simulink model "ECM"  (R2021b)
settings: Solver=VariableStepAuto  StartTime=0.0  StopTime=time(end)  RelTol=1e-3
values from neighbouring files (symbols this model uses):
  LookUpTables = struct    [LUT.m]    (also in Run_parameterestimation.m = load([Rep_Meatech, filesep,'LookUpTables_HPPC.mat']); Script_SOC_EKF.m = load('LookUpTables.mat'))
  Qnom = 2.455    [Pulse_extraction.m]    (also in Script_validation.m = 2.4162)
  SOC_init = 100    [Pulse_extraction.m]    (also in Script_SOC_EKF.m; Script_validation.m = 50)
  T_init = meas.Battery_Temp_degC(1)    [Script_validation.m]
libraries: simulink x4
settings Model: Creator=joel-louis.kone  LastModifiedBy=joel-louiskone
settings SolverCC: AlgebraicLoopSolver=TrustRegion
settings DebuggingCC: UnconnectedInputMsg=none  UnconnectedOutputMsg=none  UnconnectedLineMsg=none  SFMachineParentedDataDiag=warning
settings ModelReferenceCC: EnableRefExpFcnMdlSchedulingChecks=off

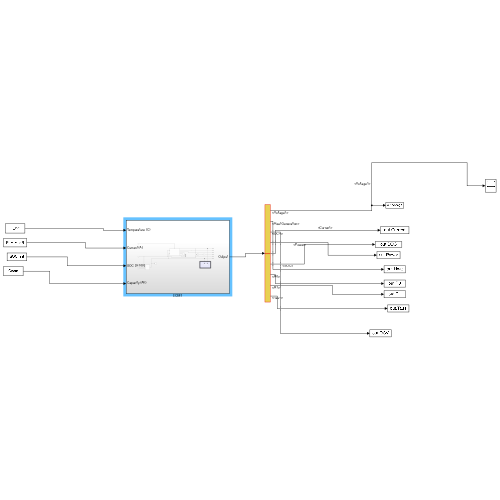
[thumbnail: Simulink's stored preview of the top-level diagram]
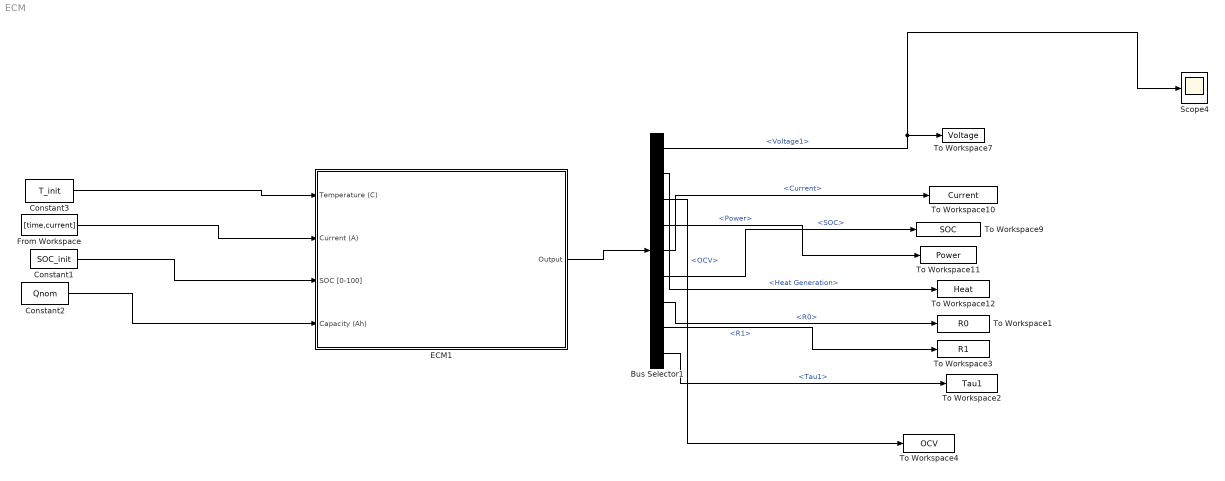
== system ECM ==
  Bus Selector1 : BusSelector  OutputSignals=Voltage1,Heat Generation,OCV,Power,Current,SOC,R0,R1,Tau1
  Constant1 : Constant  Value=SOC_init
  Constant2 : Constant  Value=Qnom
  Constant3 : Constant  Value=T_init
  ECM1 : Subsystem
  From Workspace : FromWorkspace  VariableName=[time,current]  SampleTime=0.1
  Scope4 : Scope
  To Workspace1 : ToWorkspace  VariableName=R0  SaveFormat=Structure With Time  SampleTime=-1
  To Workspace10 : ToWorkspace  VariableName=Current  SaveFormat=Structure With Time  SampleTime=-1
  To Workspace11 : ToWorkspace  VariableName=Power  SaveFormat=Structure With Time  SampleTime=-1
  To Workspace12 : ToWorkspace  VariableName=Heat  SaveFormat=Structure With Time  SampleTime=-1
  To Workspace2 : ToWorkspace  VariableName=Tau1  SaveFormat=Structure With Time  SampleTime=-1
  To Workspace3 : ToWorkspace  VariableName=R1  SaveFormat=Structure With Time  SampleTime=-1
  To Workspace4 : ToWorkspace  VariableName=OCV  SaveFormat=Structure With Time  SampleTime=-1
  To Workspace7 : ToWorkspace  VariableName=Voltage  SaveFormat=Structure With Time  SampleTime=-1
  To Workspace9 : ToWorkspace  VariableName=SOC  SaveFormat=Structure With Time  SampleTime=-1
  wires:
  Bus Selector1/5 -> To Workspace10/1  "<Current>"
  From Workspace/1 -> ECM1/2(Current (A))
  Bus Selector1/2 -> To Workspace12/1  "<Heat Generation>"
  Constant3/1 -> ECM1/1(Temperature (C))
  ECM1/1(Output) -> Bus Selector1/1
  Bus Selector1/1 -> Scope4/1, To Workspace7/1  "<Voltage1>"
  Bus Selector1/6 -> To Workspace9/1  "<SOC>"
  Bus Selector1/4 -> To Workspace11/1  "<Power>"
  Constant2/1 -> ECM1/4(Capacity (Ah))
  Constant1/1 -> ECM1/3(SOC [0-100])
  Bus Selector1/7 -> To Workspace1/1  "<R0>"
  Bus Selector1/8 -> To Workspace3/1  "<R1>"
  Bus Selector1/9 -> To Workspace2/1  "<Tau1>"
  Bus Selector1/3 -> To Workspace4/1  "<OCV>"

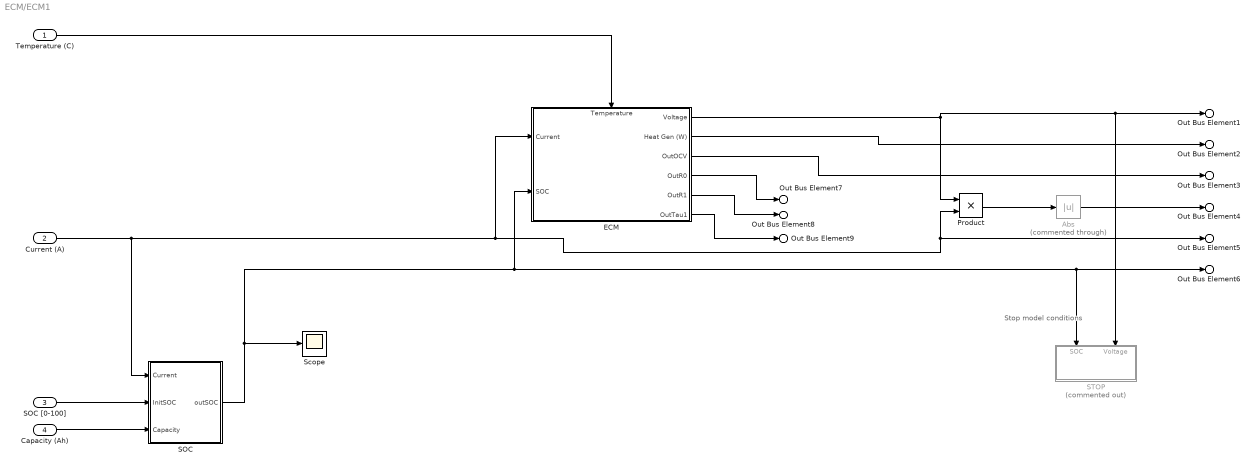
== system ECM/ECM1 ==
  note: Stop model conditions
  Temperature (C) : Inport
  Current (A) : Inport  Port=2
  SOC [0-100] : Inport  Port=3
  Capacity (Ah) : Inport  Port=4
  Abs : Abs  Commented=through
  ECM : Subsystem
      settings: PortSchema="{\"entries\":[{\"content\":{\"sides\":[{\"content\":{\"connectorIds\":[\"In1\",\"In2\"]},\"type\":\"ConnectorPlacement.EquallySpacedRectSide\",\"uuid\":\"edc5e7ae-745c-47cf-82e1-2a35e82af4f8\"},{\"content\":{\"connectorIds\":[\"Out1\",\"Out2\",\"Out3\",\"Out4\",\"Out5\",\"Out6\"],\"side\":\"RIGHT\"},\"type\":\"ConnectorPlacement.EquallySpacedRectSide\",\"uuid\":\"23604a62-cf3d-4676-b110-c126866d2dc0\"},{\"content\":{\"connectorIds\":[\"In3\"],\"side\":\"TOP\"},\"type\":\"ConnectorPlacement.EquallySpacedRectSide\",\"uuid\":\"e8176ec1-85b7-4cdd-8c72-13c05cb96821\"}]},\"type\":\"ConnectorPlacement.EquallySpacedConnector\",\"uuid\":\"8076f895-f62a-482c-9288-582d3af41eba\"}],\"packageUris\":[\"http://schema.mathworks.com/mf0/Connector/R2020b\"],\"version\":\"1.0\"}"
  Product : Product
  SOC : Subsystem
  STOP : Subsystem  Commented=on
      settings: PortSchema="{\"entries\":[{\"content\":{\"sides\":[{\"content\":{},\"type\":\"ConnectorPlacement.EquallySpacedRectSide\",\"uuid\":\"ad4b06f7-1952-4c9b-98d0-1c5b14fc528a\"},{\"content\":{\"side\":\"RIGHT\"},\"type\":\"ConnectorPlacement.EquallySpacedRectSide\",\"uuid\":\"0e87e05f-c38b-4899-9ed0-4e84cd23c8de\"},{\"content\":{\"side\":\"TOP\"},\"type\":\"ConnectorPlacement.EquallySpacedRectSide\",\"uuid\":\"e38574cc-e4d8-43c2-a247-2bbd6f40e998\"},{\"content\":{\"connectorIds\":[\"In1\",\"In2\"],\"side\":\"BOTTOM\"},\"type\":\"ConnectorPlacement.EquallySpacedRectSide\",\"uuid\":\"fa834913-df18-4dba-ad85-ee110dbadbfc\"}]},\"type\":\"ConnectorPlacement.EquallySpacedConnector\",\"uuid\":\"cbbb9c3f-18ca-424a-bd7b-42dc7388afb6\"}],\"packageUris\":[\"http://schema.mathworks.com/mf0/Connector/R2020b\"],\"version\":\"1.0\"}"
  Scope : Scope
  Out Bus Element1 : Outport  PortName=Output  Element=Voltage1
  Out Bus Element2 : Outport  PortName=Output  Element=Heat Generation
  Out Bus Element3 : Outport  PortName=Output  Element=OCV
  Out Bus Element4 : Outport  PortName=Output  Element=Power
  Out Bus Element5 : Outport  PortName=Output  Element=Current
  Out Bus Element6 : Outport  PortName=Output  Element=SOC
  Out Bus Element7 : Outport  PortName=Output  Element=R0
  Out Bus Element8 : Outport  PortName=Output  Element=R1
  Out Bus Element9 : Outport  PortName=Output  Element=Tau1
  wires:
  SOC [0-100]/1 -> SOC/2(InitSOC)
  Current (A)/1 -> Product/2, Out Bus Element5/1, ECM/1(Current), SOC/1(Current)
  ECM/2(Heat Gen (W)) -> Out Bus Element2/1
  ECM/1(Voltage) -> Product/1, Out Bus Element1/1, STOP/1(Voltage)
  Capacity (Ah)/1 -> SOC/3(Capacity)
  ECM/3(OutOCV) -> Out Bus Element3/1
  Product/1 -> Abs/1
  Abs/1 -> Out Bus Element4/1
  Temperature (C)/1 -> ECM/3(Temperature)
  SOC/1(outSOC) -> Out Bus Element6/1, STOP/2(SOC), ECM/2(SOC), Scope/1
  ECM/4(OutR0) -> Out Bus Element7/1
  ECM/5(OutR1) -> Out Bus Element8/1
  ECM/6(OutTau1) -> Out Bus Element9/1

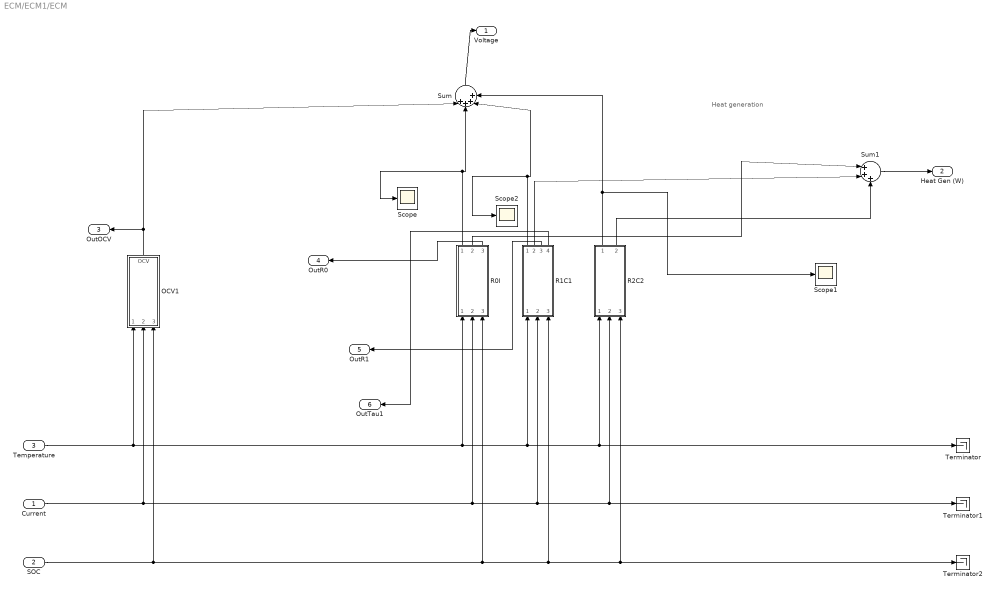
== system ECM/ECM1/ECM ==
  note: Heat generation
  Current : Inport
  SOC : Inport  Port=2
  Temperature : Inport  Port=3
  OCV1 : Subsystem
  R0I : Subsystem
  R1C1 : Subsystem
  R2C2 : Subsystem
  Scope : Scope
  Scope1 : Scope
  Scope2 : Scope
  Sum : Sum  Inputs=|++++
  Sum1 : Sum  Inputs=|+++
  Terminator : Terminator
  Terminator1 : Terminator
  Terminator2 : Terminator
  Voltage : Outport
  Heat Gen (W) : Outport  Port=2
  OutOCV : Outport  Port=3
  OutR0 : Outport  Port=4
  OutR1 : Outport  Port=5
  OutTau1 : Outport  Port=6
  wires:
  OCV1/1(OCV) -> OutOCV/1, Sum/1
  R0I/1(IRo) -> Sum/2, Scope/1
  R1C1/1(UR1C1) -> Sum/3, Scope2/1
  Sum/1 -> Voltage/1
  R2C2/1(UR2C2) -> Scope1/1, Sum/4
  R0I/2(Heat R0) -> Sum1/1
  R1C1/2(Heat R1C1) -> Sum1/2
  R2C2/2(Heat R2C2) -> Sum1/3
  Sum1/1 -> Heat Gen (W)/1
  Temperature/1 -> OCV1/1(Temperature), R0I/1(Temperature), R1C1/1(Temperature), R2C2/1(Temperature), Terminator/1
  Current/1 -> OCV1/2(Current), R1C1/2(Current), R2C2/2(Current), Terminator1/1, R0I/2(Current)
  SOC/1 -> OCV1/3(SOC), Terminator2/1, R2C2/3(SOC), R1C1/3(SOC), R0I/3(SOC)
  R0I/3(outR0) -> OutR0/1
  R1C1/3(OutR1) -> OutR1/1
  R1C1/4(OutTau1) -> OutTau1/1

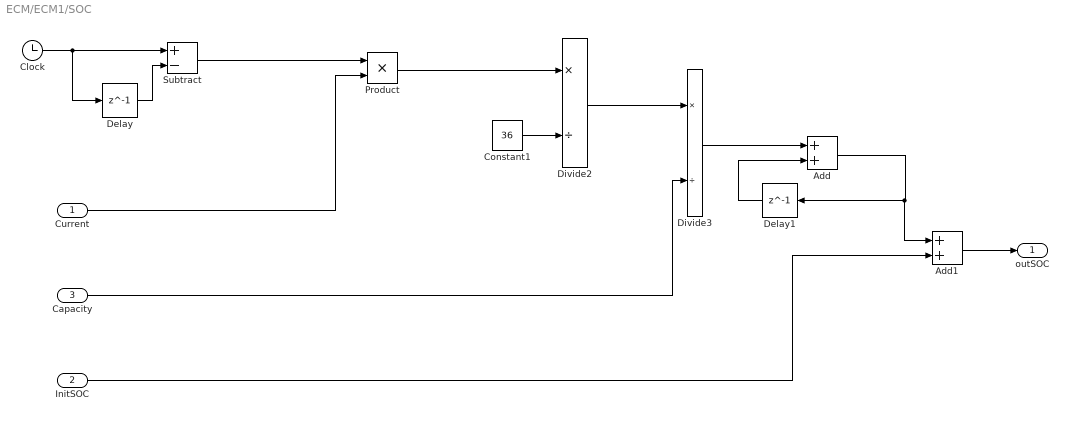
== system ECM/ECM1/SOC ==
  Current : Inport
  InitSOC : Inport  Port=2
  Capacity : Inport  Port=3
  Add : Sum
  Add1 : Sum
  Clock : Clock
  Constant1 : Constant  Value=36
  Delay : Delay  DelayLength=1
  Delay1 : Delay  DelayLength=1
  Divide2 : Product  Inputs=*/
  Divide3 : Product  Inputs=*/
  Product : Product
  Subtract : Sum  Inputs=+-
  outSOC : Outport
  wires:
  Current/1 -> Product/2
  InitSOC/1 -> Add1/2
  Delay/1 -> Subtract/2
  Clock/1 -> Subtract/1, Delay/1
  Subtract/1 -> Product/1
  Constant1/1 -> Divide2/2
  Product/1 -> Divide2/1
  Divide2/1 -> Divide3/1
  Divide3/1 -> Add/1
  Delay1/1 -> Add/2
  Add/1 -> Add1/1, Delay1/1
  Add1/1 -> outSOC/1
  Capacity/1 -> Divide3/2

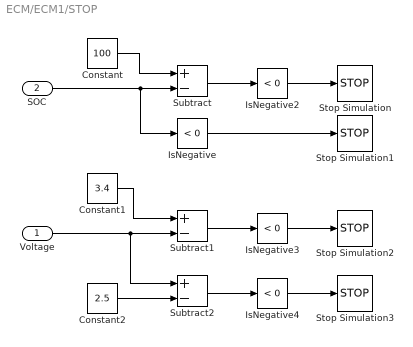
== system ECM/ECM1/STOP ==
  Voltage : Inport
  SOC : Inport  Port=2
  Constant : Constant  Value=100
  Constant1 : Constant  Value=3.4
  Constant2 : Constant  Value=2.5
  IsNegative{,2..4} (4 alike) : simulink/Logic and Bit Operations/Compare To Zero  relop=<  OutDataTypeStr=boolean
  Stop Simulation{,1..3} (4 alike) : Stop
  Subtract : Sum  Inputs=+-
  Subtract1 : Sum  Inputs=+-
  Subtract2 : Sum  Inputs=+-
  wires:
  SOC/1 -> IsNegative/1, Subtract/2
  Constant/1 -> Subtract/1
  Subtract/1 -> IsNegative2/1
  IsNegative2/1 -> Stop Simulation/1
  IsNegative/1 -> Stop Simulation1/1
  Subtract1/1 -> IsNegative3/1
  Constant1/1 -> Subtract1/1
  Voltage/1 -> Subtract2/1, Subtract1/2
  IsNegative3/1 -> Stop Simulation2/1
  Constant2/1 -> Subtract2/2
  Subtract2/1 -> IsNegative4/1
  IsNegative4/1 -> Stop Simulation3/1

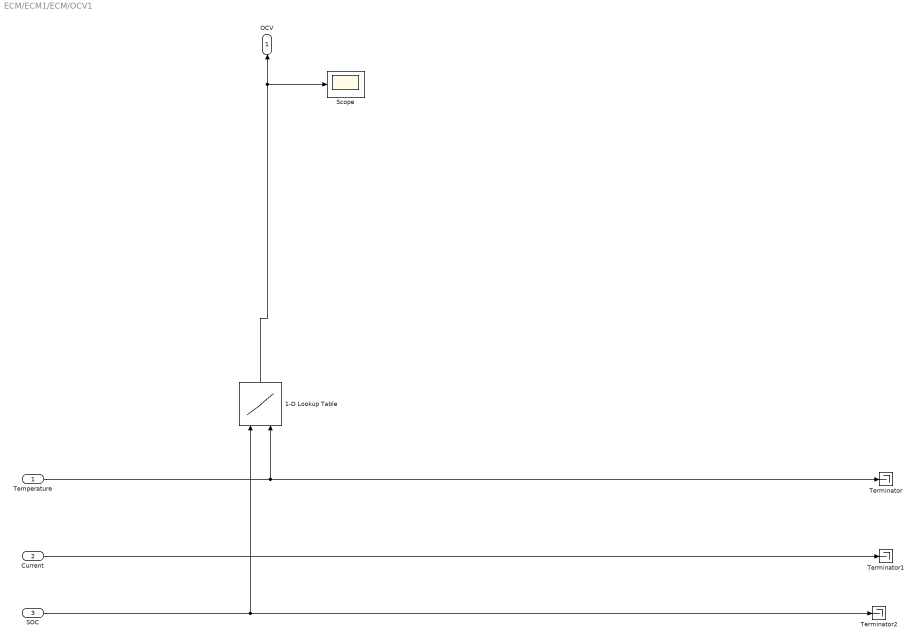
== system ECM/ECM1/ECM/OCV1 ==
  Temperature : Inport
  Current : Inport  Port=2
  SOC : Inport  Port=3
  1-D Lookup Table : Lookup_n-D  BreakpointsForDimension1=LookUpTables.OCV_SOCs  BreakpointsForDimension2=LookUpTables.OCV_Temps  BeginIndexSearchUsingPreviousIndexResult=on  Table=LookUpTables.OCV  InterpMethod=Cubic spline  ExtrapMethod=Clip  InternalRulePriority=Speed  RndMeth=Simplest  InputSameDT=on
      settings: InputPortMap=u0,u1
  Scope : Scope
  Terminator : Terminator
  Terminator1 : Terminator
  Terminator2 : Terminator
  OCV : Outport
  wires:
  Temperature/1 -> 1-D Lookup Table/2, Terminator/1
  SOC/1 -> 1-D Lookup Table/1, Terminator2/1
  Current/1 -> Terminator1/1
  1-D Lookup Table/1 -> Scope/1, OCV/1
  ? -> ?

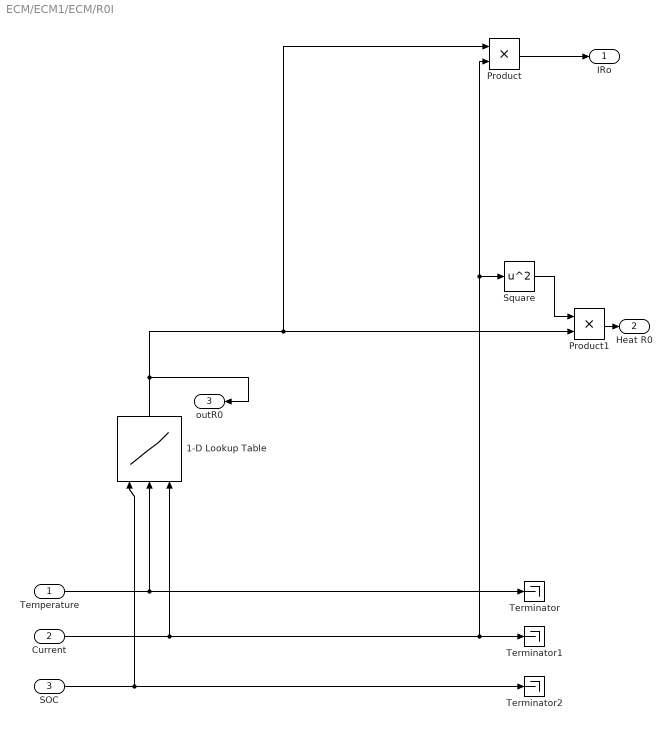
== system ECM/ECM1/ECM/R0I ==
  Temperature : Inport
  Current : Inport  Port=2
  SOC : Inport  Port=3
  1-D Lookup Table : Lookup_n-D  NumberOfTableDimensions=3  BreakpointsForDimension1=LookUpTables.SOCs  BreakpointsForDimension2=LookUpTables.Temps  BreakpointsForDimension3=LookUpTables.Crates*Qnom  BeginIndexSearchUsingPreviousIndexResult=on  Table=LookUpTables.R0  ExtrapMethod=Clip  UseLastTableValue=on  InternalRulePriority=Speed  RndMeth=Simplest  InputSameDT=on
      settings: InputPortMap=u0,u1,u2
  Product : Product
  Product1 : Product
  Square : Math  Operator=square  SaturateOnIntegerOverflow=on
  Terminator : Terminator
  Terminator1 : Terminator
  Terminator2 : Terminator
  IRo : Outport
  Heat R0 : Outport  Port=2
  outR0 : Outport  Port=3
  wires:
  SOC/1 -> Terminator2/1, 1-D Lookup Table/1
  Product/1 -> IRo/1
  Temperature/1 -> Terminator/1, 1-D Lookup Table/2
  Current/1 -> 1-D Lookup Table/3, Square/1, Product/2, Terminator1/1
  Square/1 -> Product1/1
  Product1/1 -> Heat R0/1
  1-D Lookup Table/1 -> outR0/1, Product/1, Product1/2

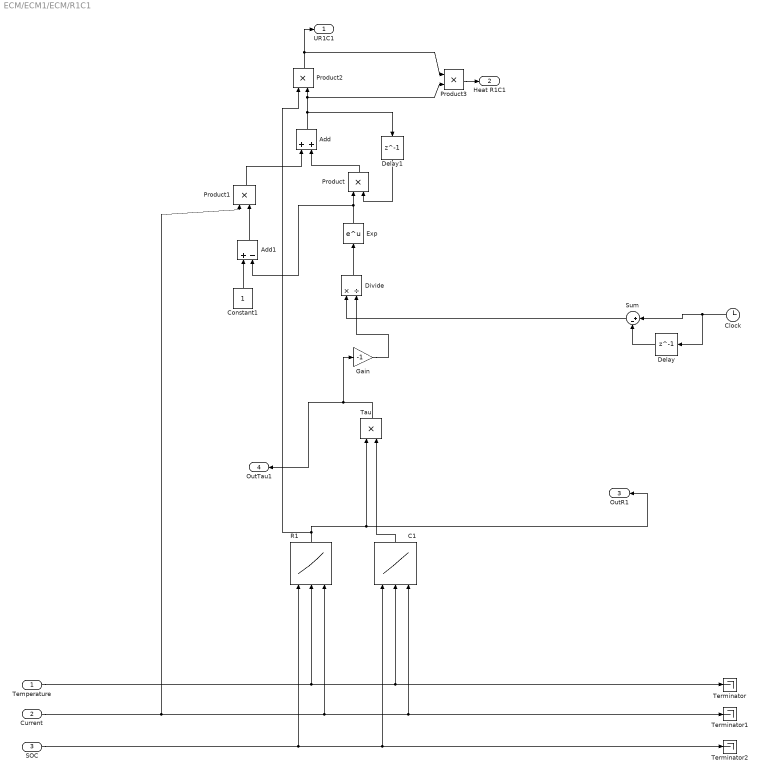
== system ECM/ECM1/ECM/R1C1 ==
  Temperature : Inport
  Current : Inport  Port=2
  SOC : Inport  Port=3
  Add : Sum
  Add1 : Sum  Inputs=+-
  C1 : Lookup_n-D  NumberOfTableDimensions=3  BreakpointsForDimension1=LookUpTables.SOCs  BreakpointsForDimension2=LookUpTables.Temps  BreakpointsForDimension3=LookUpTables.Crates*Qnom  BeginIndexSearchUsingPreviousIndexResult=on  Table=LookUpTables.C1  ExtrapMethod=Clip  UseLastTableValue=on  InternalRulePriority=Speed  RndMeth=Simplest  InputSameDT=on
      settings: InputPortMap=u0,u1,u2
  Clock : Clock
  Constant1 : Constant
  Delay : Delay  DelayLength=1
  Delay1 : Delay  DelayLength=1
  Divide : Product  Inputs=*/
  Exp : Math  SaturateOnIntegerOverflow=on
  Gain : Gain  Gain=-1
  Product{,1..3} (4 alike) : Product
  R1 : Lookup_n-D  NumberOfTableDimensions=3  BreakpointsForDimension1=LookUpTables.SOCs  BreakpointsForDimension2=LookUpTables.Temps  BreakpointsForDimension3=LookUpTables.Crates*Qnom  BeginIndexSearchUsingPreviousIndexResult=on  Table=LookUpTables.R1  ExtrapMethod=Clip  InternalRulePriority=Speed  RndMeth=Simplest  InputSameDT=on
      settings: InputPortMap=u0,u1,u2
  Sum : Sum  Inputs=|+-
  Tau : Product
  Terminator : Terminator
  Terminator1 : Terminator
  Terminator2 : Terminator
  UR1C1 : Outport
  Heat R1C1 : Outport  Port=2
  OutR1 : Outport  Port=3
  OutTau1 : Outport  Port=4
  wires:
  Temperature/1 -> Terminator/1, C1/2, R1/2
  Clock/1 -> Sum/1, Delay/1
  Delay/1 -> Sum/2
  Sum/1 -> Divide/1
  Divide/1 -> Exp/1
  Product/1 -> Add/2
  Exp/1 -> Add1/2, Product/1
  SOC/1 -> Terminator2/1, C1/1, R1/1
  R1/1 -> Product2/1, Tau/1, OutR1/1
  C1/1 -> Tau/2
  Current/1 -> R1/3, C1/3, Terminator1/1, Product1/1
  Add1/1 -> Product1/2
  Constant1/1 -> Add1/1
  Product1/1 -> Add/1
  Delay1/1 -> Product/2
  Product3/1 -> Heat R1C1/1
  Add/1 -> Product3/2, Product2/2, Delay1/1
  Product2/1 -> Product3/1, UR1C1/1
  Tau/1 -> OutTau1/1, Gain/1
  Gain/1 -> Divide/2

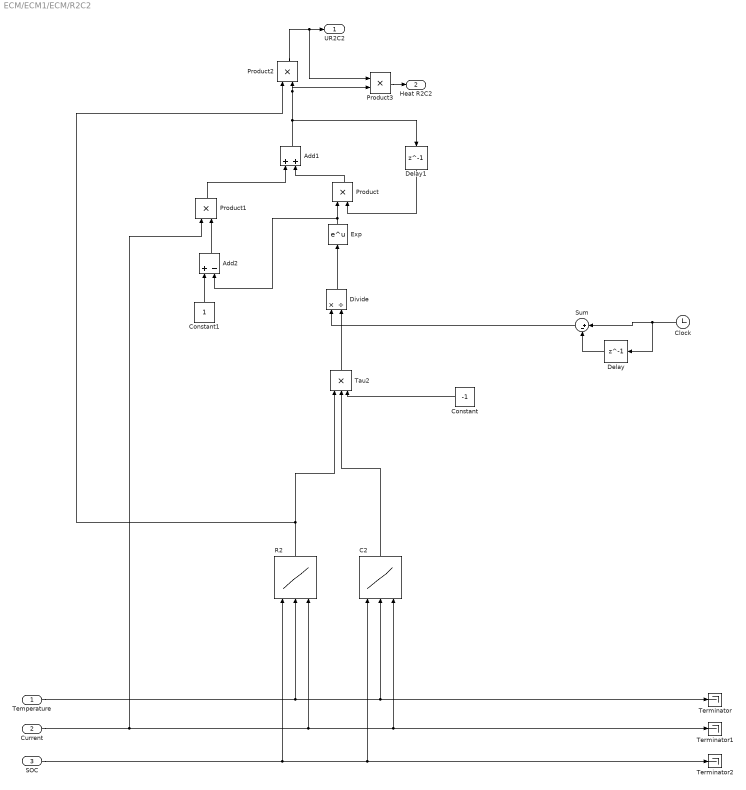
== system ECM/ECM1/ECM/R2C2 ==
  Temperature : Inport
  Current : Inport  Port=2
  SOC : Inport  Port=3
  Add1 : Sum
  Add2 : Sum  Inputs=+-
  C2 : Lookup_n-D  NumberOfTableDimensions=3  BreakpointsForDimension1=LookUpTables.SOCs  BreakpointsForDimension2=LookUpTables.Temps  BreakpointsForDimension3=LookUpTables.Crates*Qnom  BeginIndexSearchUsingPreviousIndexResult=on  Table=LookUpTables.C2  ExtrapMethod=Clip  UseLastTableValue=on  InternalRulePriority=Speed  RndMeth=Simplest  InputSameDT=on
      settings: InputPortMap=u0,u1,u2
  Clock : Clock
  Constant : Constant  Value=-1
  Constant1 : Constant
  Delay : Delay  DelayLength=1
  Delay1 : Delay  DelayLength=1
  Divide : Product  Inputs=*/
  Exp : Math  SaturateOnIntegerOverflow=on
  Product{,1..3} (4 alike) : Product
  R2 : Lookup_n-D  NumberOfTableDimensions=3  BreakpointsForDimension1=LookUpTables.SOCs  BreakpointsForDimension2=LookUpTables.Temps  BreakpointsForDimension3=LookUpTables.Crates*Qnom  BeginIndexSearchUsingPreviousIndexResult=on  Table=LookUpTables.R2  ExtrapMethod=Clip  UseLastTableValue=on  InternalRulePriority=Speed  RndMeth=Simplest  InputSameDT=on
      settings: InputPortMap=u0,u1,u2
  Sum : Sum  Inputs=|+-
  Tau2 : Product  Inputs=3
  Terminator : Terminator
  Terminator1 : Terminator
  Terminator2 : Terminator
  UR2C2 : Outport
  Heat R2C2 : Outport  Port=2
  wires:
  Clock/1 -> Delay/1, Sum/1
  Constant/1 -> Tau2/3
  Temperature/1 -> Terminator/1, C2/2, R2/2
  SOC/1 -> Terminator2/1, C2/1, R2/1
  Tau2/1 -> Divide/2
  Delay/1 -> Sum/2
  Sum/1 -> Divide/1
  Divide/1 -> Exp/1
  R2/1 -> Product2/1, Tau2/1
  C2/1 -> Tau2/2
  Product/1 -> Add1/2
  Add2/1 -> Product1/2
  Exp/1 -> Add2/2, Product/1
  Current/1 -> Product1/1, R2/3, C2/3, Terminator1/1
  Product1/1 -> Add1/1
  Constant1/1 -> Add2/1
  Delay1/1 -> Product/2
  Add1/1 -> Product3/2, Product2/2, Delay1/1
  Product2/1 -> Product3/1, UR2C2/1
  Product3/1 -> Heat R2C2/1
